simulink model "SystemWithObservers"  (R2023a)
settings: Solver=VariableStepAuto  StartTime=0.0  StopTime=100  MaxStep=0.01  RelTol=1e-3
undefined symbols (not defined in the file): DemoControllers
settings Model: Creator=andriyanov_ilya  LastModifiedBy=KozlovM

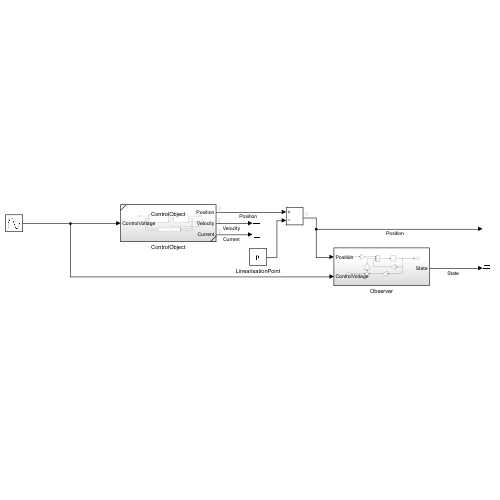
[thumbnail: Simulink's stored preview of the top-level diagram]
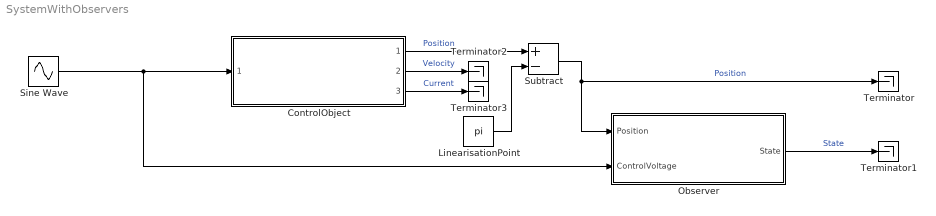
== system SystemWithObservers ==
  ControlObject : Subsystem  ReferencedSubsystem=ControlObject
  LinearisationPoint : Constant  Value=pi
  Observer : Subsystem
  Sine Wave : Sin  Amplitude=5  SampleTime=0
  Subtract : Sum  Inputs=+-
  Terminator{,1..3} (4 alike) : Terminator
  wires:
  Sine Wave/1 -> ControlObject/1, Observer/2(ControlVoltage)
  ControlObject/1 -> Subtract/1  "Position"
  LinearisationPoint/1 -> Subtract/2
  Subtract/1 -> Observer/1(Position), Terminator/1  "Position"
  Observer/1(State) -> Terminator1/1  "State"
  ControlObject/2 -> Terminator2/1  "Velocity"
  ControlObject/3 -> Terminator3/1  "Current"

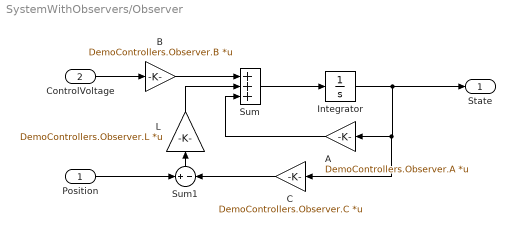
== system SystemWithObservers/Observer ==
  Position : Inport
  ControlVoltage : Inport  Port=2
  A : Gain  Gain=DemoControllers.Observer.A  Multiplication=Matrix(K*u)
  B : Gain  Gain=DemoControllers.Observer.B  Multiplication=Matrix(K*u)
  C : Gain  Gain=DemoControllers.Observer.C  Multiplication=Matrix(K*u)
  Integrator : Integrator
  L : Gain  Gain=DemoControllers.Observer.L  Multiplication=Matrix(K*u)
  Sum : Sum  Inputs=+++
  Sum1 : Sum  Inputs=+|-
  State : Outport
  wires:
  ControlVoltage/1 -> B/1
  B/1 -> Sum/1
  Sum/1 -> Integrator/1
  A/1 -> Sum/3
  Integrator/1 -> C/1, A/1, State/1
  Position/1 -> Sum1/1
  C/1 -> Sum1/2
  Sum1/1 -> L/1
  L/1 -> Sum/2
